simulink subsystem "VehicleElec"  (R2023a)
settings: Solver=VariableStepAuto  StartTime=0.0  StopTime=10.0  RelTol=1e-3
undefined symbols (not defined in the file): battery, cabin_T_init, vehicleThermal
libraries: fl_lib x95, nesl_utility x28, sdl_lib x8, slpidlib x3, simulink x2, EmotorLib x2, BatteryCurrentManagement x1, ee_lib x1
(part 1 of 3)
settings Model: Creator=jjha  LastModifiedBy=jjha
settings OptimizationCC: ReuseModelBlockBuffer=off

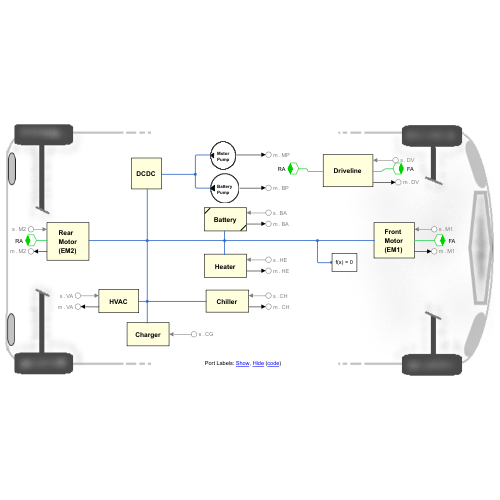
[thumbnail: Simulink's stored preview of the top-level diagram]
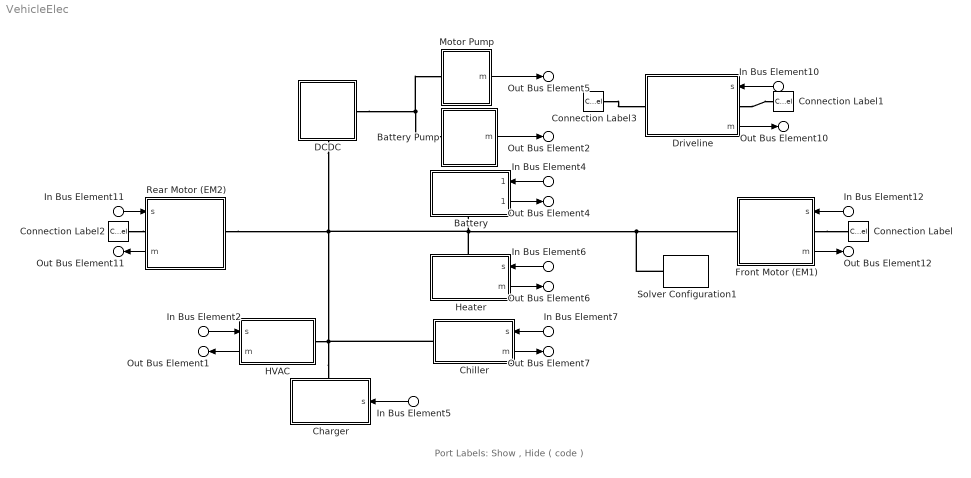
== system VehicleElec ==
  note: Port Labels: Show , Hide ( code )
  In Bus Element2 : Inport  PortName=s  Element=VA
  In Bus Element4 : Inport  PortName=s  Element=BA
  In Bus Element6 : Inport  PortName=s  Element=HE
  In Bus Element7 : Inport  PortName=s  Element=CH
  In Bus Element10 : Inport  PortName=s  Element=DV
  In Bus Element11 : Inport  PortName=s  Element=M2
  In Bus Element12 : Inport  PortName=s  Element=M1
  In Bus Element5 : Inport  PortName=s  Element=CG
  Battery : Subsystem  ReferencedSubsystem=BatteryPlantModelLumped
      settings: PortSchema="{\"entries\":[{\"content\":{\"sides\":[{\"content\":{\"connectorIds\":[\"In1\",\"Out1\"]},\"type\":\"ConnectorPlacement.EquallySpacedRectSide\",\"uuid\":\"8937d0fc-2bf4-4b6f-a857-82b384a76c94\"},{\"content\":{\"side\":\"RIGHT\"},\"type\":\"ConnectorPlacement.EquallySpacedRectSide\",\"uuid\":\"1ccbeec6-a013-4076-9f98-cb308866a19c\"},{\"content\":{\"side\":\"TOP\"},\"type\":\"ConnectorPlacement.EquallySpacedRectSide\",\"uuid\":\"77a454e3-c37c-480e-9dd0-9550186f5eb3\"},{\"content\":{\"connectorIds\":[\"RConn1\"],\"side\":\"BOTTOM\"},\"type\":\"ConnectorPlacement.EquallySpacedRectSide\",\"uuid\":\"f9a87c6a-7374-41c2-a5df-89d60c915a70\"}]},\"type\":\"ConnectorPlacement.EquallySpacedConnector\",\"uuid\":\"fe008494-fd6d-45a8-bf6b-36872afbad95\"}],\"packageUris\":[\"http://schema.mathworks.com/mf0/Connector/R2020b\"],\"version\":\"1.0\"}"
  Battery Pump : Subsystem  Tag=PublishSubsystem
      settings: PortSchema="{\"entries\":[{\"content\":{\"sides\":[{\"content\":{\"connectorIds\":[\"Out1\"]},\"type\":\"ConnectorPlacement.EquallySpacedRectSide\",\"uuid\":\"f321ff85-78a4-45a4-ab97-f20c5abfaf5e\"},{\"content\":{\"connectorIds\":[\"RConn1\"],\"side\":\"RIGHT\"},\"type\":\"ConnectorPlacement.EquallySpacedRectSide\",\"uuid\":\"2baf3540-3ef2-4140-8c68-0a1895e3ee25\"},{\"content\":{\"connectorIds\":[],\"side\":\"TOP\"},\"type\":\"ConnectorPlacement.EquallySpacedRectSide\",\"uuid\":\"1e5b09ba-71c5-41d6-b265-2fb2d783e941\"},{\"content\":{\"connectorIds\":[],\"side\":\"BOTTOM\"},\"type\":\"ConnectorPlacement.EquallySpacedRectSide\",\"uuid\":\"998b9f49-32fc-4a08-8ed4-02bb722e6368\"}]},\"type\":\"ConnectorPlacement.EquallySpacedConnector\",\"uuid\":\"4c01441a-ee4a-4858-900a-4caacc6910c3\"}],\"packageUris\":[\"http://schema.mathworks.com/mf0/Connector/R2020b\"],\"version\":\"1.0\"}"
      mask Display:
      | plot(150*cos(linspace(0, 2*pi, 500)), 150*sin(linspace(0, 2*pi, 500)))
      | patch([-100 -55 -55 -100]-50, [0 24 -24 0], [0 0 0])
      | %disp(get_param(gcb, 'Name'))
      | disp(['{\bf\fontsize{8}' get_param(gcb, 'Name') '}'], 'texmode','on');
  Charger : Subsystem
      settings: PortSchema="{\"entries\":[{\"content\":{\"sides\":[{\"content\":{\"connectorIds\":[\"In1\"]},\"type\":\"ConnectorPlacement.EquallySpacedRectSide\",\"uuid\":\"cb45011f-5d5d-4b7e-92e7-7d115d1e4fd6\"},{\"content\":{\"connectorIds\":[],\"side\":\"RIGHT\"},\"type\":\"ConnectorPlacement.EquallySpacedRectSide\",\"uuid\":\"cd67087d-6bbf-411e-9f50-cc3c1f5fce85\"},{\"content\":{\"connectorIds\":[\"LConn1\"],\"side\":\"TOP\"},\"type\":\"ConnectorPlacement.EquallySpacedRectSide\",\"uuid\":\"32ff64c9-862a-431f-9f24-2baf455cdab5\"}]},\"type\":\"ConnectorPlacement.EquallySpacedConnector\",\"uuid\":\"13ffd7d0-36a1-4766-a9dc-2d010b2a8713\"}],\"packageUris\":[\"http://schema.mathworks.com/mf0/Connector/R2020b\"],\"version\":\"1.0\"}"
      mask Display:
      | %disp(get_param(gcb, 'Name'))
      | disp(['{\bf\fontsize{12}' get_param(gcb, 'Name') '}'], 'texmode','on');
  Chiller : Subsystem
      settings: PortSchema="{\"entries\":[{\"content\":{\"sides\":[{\"content\":{\"connectorIds\":[\"LConn1\"]},\"type\":\"ConnectorPlacement.EquallySpacedRectSide\",\"uuid\":\"5c01cf01-1aa7-4ead-a658-6b31c847d37c\"},{\"content\":{\"connectorIds\":[\"In1\",\"Out1\"],\"side\":\"RIGHT\"},\"type\":\"ConnectorPlacement.EquallySpacedRectSide\",\"uuid\":\"fa598d46-0793-4efa-a9e2-c958f5dfdee6\"},{\"content\":{\"connectorIds\":[],\"side\":\"TOP\"},\"type\":\"ConnectorPlacement.EquallySpacedRectSide\",\"uuid\":\"e82d971a-2580-41ee-87fa-0ab5603b5665\"},{\"content\":{\"connectorIds\":[],\"side\":\"BOTTOM\"},\"type\":\"ConnectorPlacement.EquallySpacedRectSide\",\"uuid\":\"431a910f-738f-40ab-a4d4-f974d0793b92\"}]},\"type\":\"ConnectorPlacement.EquallySpacedConnector\",\"uuid\":\"9f63eeb1-1768-47e0-a5e5-2e43c100d3fd\"}],\"packageUris\":[\"http://schema.mathworks.com/mf0/Connector/R2020b\"],\"version\":\"1.0\"}"
      mask Display:
      | %disp(get_param(gcb, 'Name'))
      | disp(['{\bf\fontsize{12}' get_param(gcb, 'Name') '}'], 'texmode','on');
  Connection Label : ConnectionLabel  Label=FA
  Connection Label1 : ConnectionLabel  Label=FA
  Connection Label2 : ConnectionLabel  Label=RA
  Connection Label3 : ConnectionLabel  Label=RA
  DCDC : Subsystem
      settings: PortSchema="{\"entries\":[{\"content\":{\"sides\":[{\"content\":{\"connectorIds\":[]},\"type\":\"ConnectorPlacement.EquallySpacedRectSide\",\"uuid\":\"88f70306-1074-4a2f-bf6e-5266a6fad5cc\"},{\"content\":{\"connectorIds\":[\"RConn1\"],\"side\":\"RIGHT\"},\"type\":\"ConnectorPlacement.EquallySpacedRectSide\",\"uuid\":\"c9954f31-88d1-45ba-bccc-746174ca97ad\"},{\"content\":{\"connectorIds\":[],\"side\":\"TOP\"},\"type\":\"ConnectorPlacement.EquallySpacedRectSide\",\"uuid\":\"3d242faa-6d27-4f03-9691-d9501eee9202\"},{\"content\":{\"connectorIds\":[\"RConn2\"],\"side\":\"BOTTOM\"},\"type\":\"ConnectorPlacement.EquallySpacedRectSide\",\"uuid\":\"dbc5cd88-c0c4-43cc-b68d-d7b9b93e8ccf\"}]},\"type\":\"ConnectorPlacement.EquallySpacedConnector\",\"uuid\":\"8b73b678-f81c-41f4-a7f6-152147edfd1f\"}],\"packageUris\":[\"http://schema.mathworks.com/mf0/Connector/R2020b\"],\"version\":\"1.0\"}"
      mask Display:
      | %disp(get_param(gcb, 'Name'))
      | disp(['{\bf\fontsize{12}' get_param(gcb, 'Name') '}'], 'texmode','on');
  Driveline : Subsystem
      settings: PortSchema="{\"entries\":[{\"content\":{\"sides\":[{\"content\":{\"connectorIds\":[\"In1\",\"LConn1\",\"Out1\"]},\"type\":\"ConnectorPlacement.EquallySpacedRectSide\",\"uuid\":\"f321ff85-78a4-45a4-ab97-f20c5abfaf5e\"},{\"content\":{\"connectorIds\":[\"RConn1\"],\"side\":\"RIGHT\"},\"type\":\"ConnectorPlacement.EquallySpacedRectSide\",\"uuid\":\"2baf3540-3ef2-4140-8c68-0a1895e3ee25\"},{\"content\":{\"connectorIds\":[],\"side\":\"TOP\"},\"type\":\"ConnectorPlacement.EquallySpacedRectSide\",\"uuid\":\"1e5b09ba-71c5-41d6-b265-2fb2d783e941\"}]},\"type\":\"ConnectorPlacement.EquallySpacedConnector\",\"uuid\":\"4c01441a-ee4a-4858-900a-4caacc6910c3\"}],\"packageUris\":[\"http://schema.mathworks.com/mf0/Connector/R2020b\"],\"version\":\"1.0\"}"
      mask Display:
      | %disp(get_param(gcb, 'Name'))
      | disp(['{\bf\fontsize{12}' get_param(gcb, 'Name') '}'], 'texmode','on');
  Front Motor (EM1) : Subsystem
      settings: PortSchema="{\"entries\":[{\"content\":{\"sides\":[{\"content\":{\"connectorIds\":[\"In1\",\"LConn1\",\"Out1\"]},\"type\":\"ConnectorPlacement.EquallySpacedRectSide\",\"uuid\":\"7243fc6e-711d-4968-986e-a6ac860e50c1\"},{\"content\":{\"connectorIds\":[\"RConn1\"],\"side\":\"RIGHT\"},\"type\":\"ConnectorPlacement.EquallySpacedRectSide\",\"uuid\":\"18479f7a-8f27-458a-ae71-b38762574ae4\"},{\"content\":{\"connectorIds\":[],\"side\":\"TOP\"},\"type\":\"ConnectorPlacement.EquallySpacedRectSide\",\"uuid\":\"aa936f76-6865-41c5-8414-293bd7d656ce\"},{\"content\":{\"connectorIds\":[],\"side\":\"BOTTOM\"},\"type\":\"ConnectorPlacement.EquallySpacedRectSide\",\"uuid\":\"336e35a4-9a9a-4631-a8f5-a4d8b8cf9e70\"}]},\"type\":\"ConnectorPlacement.EquallySpacedConnector\",\"uuid\":\"faab3502-7b69-46ce-a6d2-3155f4c3b486\"}],\"packageUris\":[\"http://schema.mathworks.com/mf0/Connector/R2020b\"],\"version\":\"1.0\"}"
      mask Display:
      | %disp(get_param(gcb, 'Name'))
      | disp(['{\bf\fontsize{12}' get_param(gcb, 'Name') '}'], 'texmode','on');
  HVAC : Subsystem
      settings: PortSchema="{\"entries\":[{\"content\":{\"sides\":[{\"content\":{\"connectorIds\":[\"LConn1\"]},\"type\":\"ConnectorPlacement.EquallySpacedRectSide\",\"uuid\":\"f3199610-b7b9-4772-9d43-f46decbe6ee9\"},{\"content\":{\"connectorIds\":[\"In1\",\"Out1\"],\"side\":\"RIGHT\"},\"type\":\"ConnectorPlacement.EquallySpacedRectSide\",\"uuid\":\"92399d3a-435b-4545-8fb9-2408b0c62154\"},{\"content\":{\"connectorIds\":[],\"side\":\"TOP\"},\"type\":\"ConnectorPlacement.EquallySpacedRectSide\",\"uuid\":\"9d5257be-bcde-46da-a005-cbe35149e50d\"},{\"content\":{\"connectorIds\":[],\"side\":\"BOTTOM\"},\"type\":\"ConnectorPlacement.EquallySpacedRectSide\",\"uuid\":\"da7f19de-1e57-4fc2-b5c3-4c1d680ac086\"}]},\"type\":\"ConnectorPlacement.EquallySpacedConnector\",\"uuid\":\"aa27bbb1-a774-4836-83ea-faf9e12779cd\"}],\"packageUris\":[\"http://schema.mathworks.com/mf0/Connector/R2020b\"],\"version\":\"1.0\"}"
      mask Display:
      | %disp(get_param(gcb, 'Name'))
      | disp(['{\bf\fontsize{12}' get_param(gcb, 'Name') '}'], 'texmode','on');
  Heater : Subsystem
      settings: PortSchema="{\"entries\":[{\"content\":{\"sides\":[{\"content\":{\"connectorIds\":[]},\"type\":\"ConnectorPlacement.EquallySpacedRectSide\",\"uuid\":\"f321ff85-78a4-45a4-ab97-f20c5abfaf5e\"},{\"content\":{\"connectorIds\":[\"RConn1\"],\"side\":\"RIGHT\"},\"type\":\"ConnectorPlacement.EquallySpacedRectSide\",\"uuid\":\"2baf3540-3ef2-4140-8c68-0a1895e3ee25\"},{\"content\":{\"connectorIds\":[\"Out1\",\"In1\"],\"side\":\"TOP\"},\"type\":\"ConnectorPlacement.EquallySpacedRectSide\",\"uuid\":\"1e5b09ba-71c5-41d6-b265-2fb2d783e941\"},{\"content\":{\"connectorIds\":[],\"side\":\"BOTTOM\"},\"type\":\"ConnectorPlacement.EquallySpacedRectSide\",\"uuid\":\"2993c442-350f-4391-ac34-e98798b669d5\"}]},\"type\":\"ConnectorPlacement.EquallySpacedConnector\",\"uuid\":\"4c01441a-ee4a-4858-900a-4caacc6910c3\"}],\"packageUris\":[\"http://schema.mathworks.com/mf0/Connector/R2020b\"],\"version\":\"1.0\"}"
      mask Display:
      | %disp(get_param(gcb, 'Name'))
      | disp(['{\bf\fontsize{12}' get_param(gcb, 'Name') '}'], 'texmode','on');
  Motor Pump : Subsystem  Tag=PublishSubsystem
      settings: PortSchema="{\"entries\":[{\"content\":{\"sides\":[{\"content\":{\"connectorIds\":[\"Out1\"]},\"type\":\"ConnectorPlacement.EquallySpacedRectSide\",\"uuid\":\"dafa5c41-979f-4f2b-beb0-03378b6030c3\"},{\"content\":{\"connectorIds\":[\"RConn1\"],\"side\":\"RIGHT\"},\"type\":\"ConnectorPlacement.EquallySpacedRectSide\",\"uuid\":\"2ea2b4cc-bcb0-4b93-915b-9928efecd2a3\"},{\"content\":{\"connectorIds\":[],\"side\":\"TOP\"},\"type\":\"ConnectorPlacement.EquallySpacedRectSide\",\"uuid\":\"e510a9c0-a763-4750-a71a-9698d7ffd631\"},{\"content\":{\"connectorIds\":[],\"side\":\"BOTTOM\"},\"type\":\"ConnectorPlacement.EquallySpacedRectSide\",\"uuid\":\"6a9cd967-74c4-4a03-9c08-7c7b4b09ecc0\"}]},\"type\":\"ConnectorPlacement.EquallySpacedConnector\",\"uuid\":\"4a878def-b7f5-448f-823c-c871001bb196\"}],\"packageUris\":[\"http://schema.mathworks.com/mf0/Connector/R2020b\"],\"version\":\"1.0\"}"
      mask Display:
      | plot(150*cos(linspace(0, 2*pi, 500)), 150*sin(linspace(0, 2*pi, 500)))
      | patch([-100 -55 -55 -100]-50, [0 24 -24 0], [0 0 0])
      | %disp(get_param(gcb, 'Name'))
      | disp(['{\bf\fontsize{8}' get_param(gcb, 'Name') '}'], 'texmode','on');
  Rear Motor (EM2) : Subsystem
      settings: PortSchema="{\"entries\":[{\"content\":{\"sides\":[{\"content\":{\"connectorIds\":[\"LConn1\"]},\"type\":\"ConnectorPlacement.EquallySpacedRectSide\",\"uuid\":\"50b93907-dab5-4c80-8f3d-b9696f7ba561\"},{\"content\":{\"connectorIds\":[\"In1\",\"RConn1\",\"Out1\"],\"side\":\"RIGHT\"},\"type\":\"ConnectorPlacement.EquallySpacedRectSide\",\"uuid\":\"ca5b0fd2-80b7-4a93-a409-39e052d42ed0\"},{\"content\":{\"connectorIds\":[],\"side\":\"TOP\"},\"type\":\"ConnectorPlacement.EquallySpacedRectSide\",\"uuid\":\"a20c906c-aee3-4b84-9c3f-344dbfe549ed\"},{\"content\":{\"connectorIds\":[],\"side\":\"BOTTOM\"},\"type\":\"ConnectorPlacement.EquallySpacedRectSide\",\"uuid\":\"c8c8c4b4-9dd9-46bd-a7c0-676d6e20cefe\"}]},\"type\":\"ConnectorPlacement.EquallySpacedConnector\",\"uuid\":\"5e07fad4-8c29-4119-b1ea-c96ebc59433e\"}],\"packageUris\":[\"http://schema.mathworks.com/mf0/Connector/R2020b\"],\"version\":\"1.0\"}"
      mask Display:
      | %disp(get_param(gcb, 'Name'))
      | disp(['{\bf\fontsize{12}' get_param(gcb, 'Name') '}'], 'texmode','on');
  Solver Configuration1 : nesl_utility/Solver Configuration  PhysicalDomain=network_engine_domain  SubClassName=solver  LeftPortType=input  RightPortType=generic  Tones=[]  Harmonics=[]  SimulateNoise=off  Profile=off  UseLocalSampling=off  EnableSwitchedLinearOptims=on  FrequencyDomain=off  UseCCode=off  RelTol=0.001  AbsTol=0.001  MinStep=1e-09  ToWorkspace=off  RevertToSquareIcSolve=off  NumHomotopyIterations=100  PhasorMode=off  PhasorModeNumHarmonics=1  ConsistencySolver=NEWTON_XTOL_AFTER_FTOL  IndexReductionMethod=DerivativeReplacement  DoDC=off  ResidualTolerance=1e-09  ConsistencyTolSource=GLOBAL  ConsistencyAbsTol=0.001  ConsistencyRelTol=0.001  ConsistencyTolFactor=0.001  UseLocalSolver=off  LocalSolverChoice=NE_BACKWARD_EULER_ADVANCER  ResolveIndetEquations=on  FunctionEvalNumThread=1  LocalSolverSampleTime=0.001  DoFixedCost=off  MaxNonlinIter=3  MaxModeIter=2  ComputeImpulses=off  ImpulseIterations=2  LinearAlgebra=auto  LinearAlgebraNumThread=0  EquationFormulation=NE_TIME_EF  DelaysMemoryBudget=1024  AutomaticFiltering=on  FilteringTimeConstant=0.001  PartitionStorageMethod=AS_NEEDED  PartitionMemoryBudget=1024  PartitionMethod=ROBUST
  Out Bus Element1 : Outport  PortName=m  Element=VA
  Out Bus Element4 : Outport  PortName=m  Element=BA
  Out Bus Element6 : Outport  PortName=m  Element=HE
  Out Bus Element7 : Outport  PortName=m  Element=CH
  Out Bus Element10 : Outport  PortName=m  Element=DV
  Out Bus Element11 : Outport  PortName=m  Element=M2
  Out Bus Element12 : Outport  PortName=m  Element=M1
  Out Bus Element5 : Outport  PortName=m  Element=MP
  Out Bus Element2 : Outport  PortName=m  Element=BP
  wires:
  In Bus Element2/1 -> HVAC/1(s)
  In Bus Element6/1 -> Heater/1(s)
  In Bus Element4/1 -> Battery/1
  Chiller/1(m) -> Out Bus Element7/1
  In Bus Element7/1 -> Chiller/1(s)
  Battery/1 -> Out Bus Element4/1
  HVAC/1(m) -> Out Bus Element1/1
  Driveline/1(m) -> Out Bus Element10/1
  In Bus Element10/1 -> Driveline/1(s)
  In Bus Element11/1 -> Rear Motor (EM2)/1(s)
  Rear Motor (EM2)/1(m) -> Out Bus Element11/1
  In Bus Element12/1 -> Front Motor (EM1)/1(s)
  Front Motor (EM1)/1(m) -> Out Bus Element12/1
  In Bus Element5/1 -> Charger/1(s)
  Heater/1(m) -> Out Bus Element6/1
  Motor Pump/1("  m ") -> Out Bus Element5/1
  Battery Pump/1("  m ") -> Out Bus Element2/1
  connections:
  Charger/LConn1 -- Solver Configuration1/RConn1 -- Front Motor (EM1)/RConn1 -- Heater/RConn1 -- Battery/RConn1 -- DCDC/RConn2 -- Rear Motor (EM2)/LConn1 -- HVAC/LConn1 -- Chiller/LConn1
  Battery Pump/RConn1 -- DCDC/RConn1 -- Motor Pump/RConn1
  Connection Label2/LConn1 -- Rear Motor (EM2)/RConn1
  Front Motor (EM1)/LConn1 -- Connection Label/LConn1
  Driveline/LConn1 -- Connection Label1/LConn1
  Connection Label3/LConn1 -- Driveline/RConn1

== system VehicleElec/Battery Pump ==
  Controlled Current Source : fl_lib/Electrical/Electrical Sources/Controlled Current Source
  Electrical Reference : fl_lib/Electrical/Electrical Elements/Electrical Reference
  PS Constant : fl_lib/Physical Signals/Sources/PS Constant  constant=0 A
  current sensing1 : Subsystem
      settings: PortSchema="{\"entries\":[{\"content\":{\"sides\":[{\"content\":{\"connectorIds\":[\"LConn1\"]},\"type\":\"ConnectorPlacement.EquallySpacedRectSide\",\"uuid\":\"be2815b5-7c4b-4452-9f46-9765620d338b\"},{\"content\":{\"connectorIds\":[\"RConn1\"],\"side\":\"RIGHT\"},\"type\":\"ConnectorPlacement.EquallySpacedRectSide\",\"uuid\":\"398ebab2-f4fa-4d00-bf6e-74bf1f6972c5\"},{\"content\":{\"connectorIds\":[\"Out1\"],\"side\":\"TOP\"},\"type\":\"ConnectorPlacement.EquallySpacedRectSide\",\"uuid\":\"f18d5713-17ec-4be9-9072-3e03c5a4f599\"}]},\"type\":\"ConnectorPlacement.EquallySpacedConnector\",\"uuid\":\"966ec05e-6316-4039-8e26-1d6b096cf423\"}],\"packageUris\":[\"http://schema.mathworks.com/mf0/Connector/R2020b\"],\"version\":\"1.0\"}"
  LV : PMIOPort  Side=Right
  Bus Element Out : Outport  PortName=m  Element=BattPumpCurr
  wires:
  current sensing1/1("   ") -> Bus Element Out/1  "BattPumpCurr"
  connections:
  Controlled Current Source/LConn1 -- Electrical Reference/LConn1
  PS Constant/RConn1 -- Controlled Current Source/RConn1
  current sensing1/RConn1 -- Controlled Current Source/RConn2
  current sensing1/LConn1 -- LV/RConn1

== system VehicleElec/Charger ==
  s : Inport
  Battery CC-CV : BatteryCurrentManagement/Battery CC-CV  MaxCellVoltage=battery.ChargeMaxVolt  Kp=battery.ChargeKp  Ki=battery.ChargerKi  Kaw=battery.ChargerKaw  Kt=1  Ts=-1
      settings: LibrarySourceBlock=batt_sl_lib/Current Management/Battery CC-CV
  Bus Selector4 : BusSelector  OutputSignals=Batt.Relay.RelayChg,Batt.BattSensor.CellVoltMax
  Constant Chg Current : Constant  Value=battery.ChargerCC_A
  Controlled Current Source : fl_lib/Electrical/Electrical Sources/Controlled Current Source
  Electrical Reference : fl_lib/Electrical/Electrical Elements/Electrical Reference
  Ground : Ground
  Simulink-PS Converter1 : nesl_utility/Simulink-PS Converter  PhysicalDomain=network_engine_domain  SubClassName=ps_input  LeftPortType=input  RightPortType=output  PseudoPeriodic=off  Frequencies=[]  NoiseDistribution=none  NoiseParameters=[]  Unit=A  AffineConversion=off  FilteringAndDerivatives=filter  SimscapeFilterOrder=2  InputFilterTimeConstant=0.01  UdotUserProvided=0
  Transfer Fcn : TransferFcn  Denominator=[1 1]
  HV : PMIOPort  Side=Left
  wires:
  Transfer Fcn/1 -> Simulink-PS Converter1/1
  Constant Chg Current/1 -> Battery CC-CV/3
  Bus Selector4/2 -> Battery CC-CV/2  "<CellVoltMax>"
  Bus Selector4/1 -> Battery CC-CV/1  "<RelayChg>"
  Battery CC-CV/1 -> Transfer Fcn/1
  Ground/1 -> Battery CC-CV/4
  s/1 -> Bus Selector4/1
  connections:
  Electrical Reference/LConn1 -- Controlled Current Source/RConn2
  HV/RConn1 -- Controlled Current Source/LConn1
  Controlled Current Source/RConn1 -- Simulink-PS Converter1/RConn1

== system VehicleElec/Chiller ==
  s : Inport
  Bus Selector : BusSelector  OutputSignals=Batt.BatSt,cmdChillerByp
  Chiller Subsystem : Subsystem
      settings: PortSchema="{\"entries\":[{\"content\":{\"sides\":[{\"content\":{\"connectorIds\":[\"LConn1\",\"In1\",\"In2\"]},\"type\":\"ConnectorPlacement.EquallySpacedRectSide\",\"uuid\":\"d995acd0-973b-4873-b050-eaa71c2c53f5\"},{\"content\":{\"connectorIds\":[\"RConn1\",\"RConn2\"],\"side\":\"RIGHT\"},\"type\":\"ConnectorPlacement.EquallySpacedRectSide\",\"uuid\":\"f40dc2d9-a9a2-427c-8e3f-65ba63c73559\"},{\"content\":{\"connectorIds\":[],\"side\":\"TOP\"},\"type\":\"ConnectorPlacement.EquallySpacedRectSide\",\"uuid\":\"1868aaf5-b9f5-4fdb-94e9-4b9189d403a5\"}]},\"type\":\"ConnectorPlacement.EquallySpacedConnector\",\"uuid\":\"c13a0ccf-549d-47cf-8e66-a96ce55255c8\"}],\"packageUris\":[\"http://schema.mathworks.com/mf0/Connector/R2020b\"],\"version\":\"1.0\"}"
  Controlled Current Source : fl_lib/Electrical/Electrical Sources/Controlled Current Source
  Electrical Reference : fl_lib/Electrical/Electrical Elements/Electrical Reference
  Electrical Reference1 : fl_lib/Electrical/Electrical Elements/Electrical Reference
  PS Terminator : fl_lib/Physical Signals/Sinks/PS Terminator
  Voltage Sensor : fl_lib/Electrical/Electrical Sensors/Voltage Sensor
  current sensing1 : Subsystem
      settings: PortSchema="{\"entries\":[{\"content\":{\"sides\":[{\"content\":{\"connectorIds\":[\"LConn1\"]},\"type\":\"ConnectorPlacement.EquallySpacedRectSide\",\"uuid\":\"be2815b5-7c4b-4452-9f46-9765620d338b\"},{\"content\":{\"connectorIds\":[\"RConn1\"],\"side\":\"RIGHT\"},\"type\":\"ConnectorPlacement.EquallySpacedRectSide\",\"uuid\":\"398ebab2-f4fa-4d00-bf6e-74bf1f6972c5\"},{\"content\":{\"connectorIds\":[\"Out1\"],\"side\":\"TOP\"},\"type\":\"ConnectorPlacement.EquallySpacedRectSide\",\"uuid\":\"f18d5713-17ec-4be9-9072-3e03c5a4f599\"}]},\"type\":\"ConnectorPlacement.EquallySpacedConnector\",\"uuid\":\"966ec05e-6316-4039-8e26-1d6b096cf423\"}],\"packageUris\":[\"http://schema.mathworks.com/mf0/Connector/R2020b\"],\"version\":\"1.0\"}"
  HV : PMIOPort  Side=Left
  Bus Element Out : Outport  PortName=m  Element=ChillerCurrent
  wires:
  s/1 -> Bus Selector/1
  current sensing1/1("   ") -> Bus Element Out/1  "AuxHiCurrentC"
  Bus Selector/2 -> Chiller Subsystem/2(ThCtrl)  "<cmdChillerByp>"
  Bus Selector/1 -> Chiller Subsystem/1(BattSt)  "<BatSt>"
  connections:
  Voltage Sensor/RConn1 -- Chiller Subsystem/LConn1
  Electrical Reference1/LConn1 -- Voltage Sensor/RConn2
  Controlled Current Source/RConn1 -- Chiller Subsystem/RConn1
  Controlled Current Source/LConn1 -- Electrical Reference/LConn1
  HV/RConn1 -- Voltage Sensor/LConn1 -- current sensing1/LConn1
  Controlled Current Source/RConn2 -- current sensing1/RConn1
  PS Terminator/LConn1 -- Chiller Subsystem/RConn2

== system VehicleElec/DCDC ==
  DC-DC Converter : ee_lib/Semiconductors & Converters/Converters/DC-DC Converter  Vref_option=ee.enum.converters.voltageref.internal  v_ref=100 V  P_rated=10000 W  droop_enabled=false  droop_param=ee.enum.converters.droop.value  droop=0.1 V/A  droop_percent=2  Vref_droop=10 V  reversible=ee.enum.converters.directionality.unidirectional  G_diode=1e-8 1/Ohm  P_fixed=1 W  losses_option=ee.enum.converters.lossesOption.proportionalToSquaredCurrent  eff_rated=80  tableOption=ee.enum.converters.lossTableOptionThermal.currentTemp  i_eff_vec=[-2, -1, 1, 2] A  v_eff_vec=[15, 30, 45] V  eff_vec=[66, 76, 80, 74]  eff_2D_table=[66, 66, 66; 76, 76, 76; 80, 80, 80; 74, 74, 74]  model_dynamics=ee.enum.converters.dynamics.yes  tau=0.02 s  v_ini=10 V  v1_min=1 V  R1=1000 Ohm  R2=1000 Ohm  enable_fault=simscape.enum.onoff.off  fault_condition=ee.enum.faults.faultInputCondition.greaterThan  fault_threshold=0.5  T_eff_vec=[280, 300, 320] K  eff_3D_table=repmat([66; 76; 80; 74], 1, 3, 3)  thermal_mass=100 J/K  initial_temperature=298.15 K
      settings: InternalSimscapePortConfiguration="{\"Bottom\":[],\"Left\":[{\"id\":\"p1\",\"label\":\"1+\",\"type\":\"foundation.electrical.electrical\"},{\"id\":\"n1\",\"label\":\"1-\",\"type\":\"foundation.electrical.electrical\"}],\"Right\":[{\"id\":\"p2\",\"label\":\"2+\",\"type\":\"foundation.electrical.electrical\"},{\"id\":\"n2\",\"label\":\"2-\",\"type\":\"foundation.electrical.electrical\"}],\"Top\":[]}"
  Electrical Reference : fl_lib/Electrical/Electrical Elements/Electrical Reference
  Electrical Reference1 : fl_lib/Electrical/Electrical Elements/Electrical Reference
  LV : PMIOPort  Side=Right
  HV : PMIOPort  Port=2  Side=Right
  connections:
  LV/RConn1 -- DC-DC Converter/RConn1
  Electrical Reference/LConn1 -- DC-DC Converter/RConn2
  HV/RConn1 -- DC-DC Converter/LConn1
  DC-DC Converter/LConn2 -- Electrical Reference1/LConn1

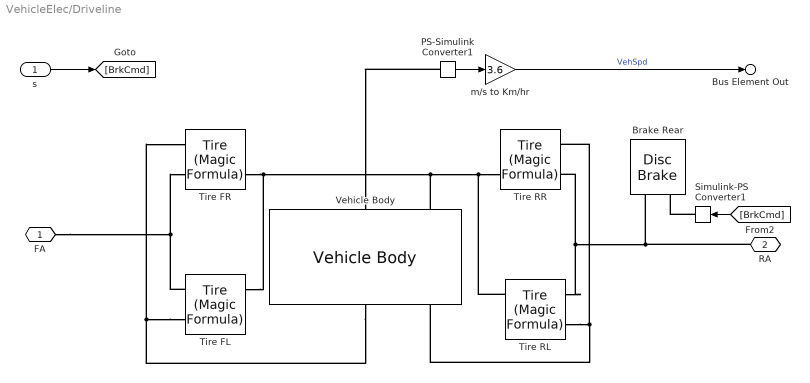
== system VehicleElec/Driveline ==
  s : Inport
  Brake Rear : sdl_lib/Brakes & Detents/Rotational/Disc Brake  r_mean=150 mm  bore=10 mm  n_pads=2  thermal_port=simscape.enum.thermaleffects.omit  mu_static=0.9  mu_coulomb=0.7  temperature_TLU=[280, 300, 320] K  mu_static_TLU=[.9, .8, .7]  mu_coulomb_TLU=[.8, .7, .6]  brkwy_vel=0.1 rad/s  visc_coef=0 N*m*s/rad  enable_faults=simscape.enum.onoff.off  faulted_pressure=0 bar  external_fault=simscape.enum.onoff.off  temporal_fault=simscape.enum.onoff.off  fault_time=5 s  report_fault=simscape.enum.assert.action.none  thermal_mass=50 kJ/K  temperature_specify=off  temperature_priority=High  temperature=300 K  temperature_nominal_specify=off  temperature_nominal_unit=K  temperature_nominal_value=1
  PS-Simulink Converter1 : nesl_utility/PS-Simulink Converter  PhysicalDomain=network_engine_domain  SubClassName=ps_output  LeftPortType=input  RightPortType=output  PseudoPeriodic=off  Frequencies=[]  VectorFormat=inherit  Unit=inherit  AffineConversion=off
  Simulink-PS Converter1 : nesl_utility/Simulink-PS Converter  PhysicalDomain=network_engine_domain  SubClassName=ps_input  LeftPortType=input  RightPortType=output  PseudoPeriodic=off  Frequencies=[]  NoiseDistribution=none  NoiseParameters=[]  Unit=1  AffineConversion=off  FilteringAndDerivatives=provide  SimscapeFilterOrder=1  InputFilterTimeConstant=0.001  UdotUserProvided=0
  Tire FL : sdl_lib/Tires & Vehicles/Tire (Magic Formula)  parameterization=sdl.enum.magic_tire_model.peak  F_z1=3000 N  F_x1=3500 N  kappa1=10  B_m=10  C_m=1.9  D_m=1  E_m=0.97  fz0=4000 N  p_Cx=1.685  p_Dx=[1.21, -.037]  p_Ex=[.344, .095, -.02, 0]  p_Kx=[21.51, -.163, .245]  p_Hx=[-.002, .002]  p_Vx=[0, 0]  rolling_radius_model=sdl.enum.RollingRadiusParameterization.Constant  r_e="vehicle.tireRollingRadius_cm  cm"  r_0=0.3 m  breff=8.39  dreff=0.26  freff=0.074  q_re0=0.99  q_v1=0.008  longvl=17 m/s  cz=5e5 N/m  model_resistance=simscape.enum.onoff.off  resistance_model=sdl.enum.rollingResistanceParameterization.constant  coeff=0.015  p_tire=250e3 Pa  alpha=-0.003  beta=0.97  coeff_a=84e-4  coeff_b=6.2e-4 s/m  coeff_c=1.6e-4 s^2/m^2  p_tire0=240e3 Pa  fz0_resistance=4000 N  vH0=16 m/s  q_Sy=[.0082, 0, .0014, .001, 0, 0, 1.08, -.5]  v_thr=0.001 m/s  enable_scaling_coefficients=false  lfzO=1  lcx=1  lmux=1  lex=1  lkx=1  lhx=1  lvx=1  lmy=1  model_compliance=sdl.enum.compliance.off  stiffness=1e6 N/m  damping=1000 N*s/m  model_inertia=sdl.enum.model_inertia.off  inertia=1 kg*m^2  initial_velocity=0 rad/s  vxlow=0.1 m/s  v_tr_thr=0.1*(0.1) m/s  kpumin=-1e5  kpumax=1e5
  Tire FR : sdl_lib/Tires & Vehicles/Tire (Magic Formula)  parameterization=sdl.enum.magic_tire_model.peak  F_z1=3000 N  F_x1=3500 N  kappa1=10  B_m=10  C_m=1.9  D_m=1  E_m=0.97  fz0=4000 N  p_Cx=1.685  p_Dx=[1.21, -.037]  p_Ex=[.344, .095, -.02, 0]  p_Kx=[21.51, -.163, .245]  p_Hx=[-.002, .002]  p_Vx=[0, 0]  rolling_radius_model=sdl.enum.RollingRadiusParameterization.Constant  r_e="vehicle.tireRollingRadius_cm  cm"  r_0=0.3 m  breff=8.39  dreff=0.26  freff=0.074  q_re0=0.99  q_v1=0.008  longvl=17 m/s  cz=5e5 N/m  model_resistance=simscape.enum.onoff.off  resistance_model=sdl.enum.rollingResistanceParameterization.constant  coeff=0.015  p_tire=250e3 Pa  alpha=-0.003  beta=0.97  coeff_a=84e-4  coeff_b=6.2e-4 s/m  coeff_c=1.6e-4 s^2/m^2  p_tire0=240e3 Pa  fz0_resistance=4000 N  vH0=16 m/s  q_Sy=[.0082, 0, .0014, .001, 0, 0, 1.08, -.5]  v_thr=0.001 m/s  enable_scaling_coefficients=false  lfzO=1  lcx=1  lmux=1  lex=1  lkx=1  lhx=1  lvx=1  lmy=1  model_compliance=sdl.enum.compliance.off  stiffness=1e6 N/m  damping=1000 N*s/m  model_inertia=sdl.enum.model_inertia.off  inertia=1 kg*m^2  initial_velocity=0 rad/s  vxlow=0.1 m/s  v_tr_thr=0.1*(0.1) m/s  kpumin=-1e5  kpumax=1e5
  Tire RL : sdl_lib/Tires & Vehicles/Tire (Magic Formula)  parameterization=sdl.enum.magic_tire_model.peak  F_z1=3000 N  F_x1=3500 N  kappa1=10  B_m=10  C_m=1.9  D_m=1  E_m=0.97  fz0=4000 N  p_Cx=1.685  p_Dx=[1.21, -.037]  p_Ex=[.344, .095, -.02, 0]  p_Kx=[21.51, -.163, .245]  p_Hx=[-.002, .002]  p_Vx=[0, 0]  rolling_radius_model=sdl.enum.RollingRadiusParameterization.Constant  r_e="vehicle.tireRollingRadius_cm  cm"  r_0=0.3 m  breff=8.39  dreff=0.26  freff=0.074  q_re0=0.99  q_v1=0.008  longvl=17 m/s  cz=5e5 N/m  model_resistance=simscape.enum.onoff.off  resistance_model=sdl.enum.rollingResistanceParameterization.constant  coeff=0.015  p_tire=250e3 Pa  alpha=-0.003  beta=0.97  coeff_a=84e-4  coeff_b=6.2e-4 s/m  coeff_c=1.6e-4 s^2/m^2  p_tire0=240e3 Pa  fz0_resistance=4000 N  vH0=16 m/s  q_Sy=[.0082, 0, .0014, .001, 0, 0, 1.08, -.5]  v_thr=0.001 m/s  enable_scaling_coefficients=false  lfzO=1  lcx=1  lmux=1  lex=1  lkx=1  lhx=1  lvx=1  lmy=1  model_compliance=sdl.enum.compliance.off  stiffness=1e6 N/m  damping=1000 N*s/m  model_inertia=sdl.enum.model_inertia.off  inertia=1 kg*m^2  initial_velocity=0 rad/s  vxlow=0.1 m/s  v_tr_thr=0.1*(0.1) m/s  kpumin=-1e5  kpumax=1e5
  Tire RR : sdl_lib/Tires & Vehicles/Tire (Magic Formula)  parameterization=sdl.enum.magic_tire_model.peak  F_z1=3000 N  F_x1=3500 N  kappa1=10  B_m=10  C_m=1.9  D_m=1  E_m=0.97  fz0=4000 N  p_Cx=1.685  p_Dx=[1.21, -.037]  p_Ex=[.344, .095, -.02, 0]  p_Kx=[21.51, -.163, .245]  p_Hx=[-.002, .002]  p_Vx=[0, 0]  rolling_radius_model=sdl.enum.RollingRadiusParameterization.Constant  r_e="vehicle.tireRollingRadius_cm  cm"  r_0=0.3 m  breff=8.39  dreff=0.26  freff=0.074  q_re0=0.99  q_v1=0.008  longvl=17 m/s  cz=5e5 N/m  model_resistance=simscape.enum.onoff.off  resistance_model=sdl.enum.rollingResistanceParameterization.constant  coeff=0.015  p_tire=250e3 Pa  alpha=-0.003  beta=0.97  coeff_a=84e-4  coeff_b=6.2e-4 s/m  coeff_c=1.6e-4 s^2/m^2  p_tire0=240e3 Pa  fz0_resistance=4000 N  vH0=16 m/s  q_Sy=[.0082, 0, .0014, .001, 0, 0, 1.08, -.5]  v_thr=0.001 m/s  enable_scaling_coefficients=false  lfzO=1  lcx=1  lmux=1  lex=1  lkx=1  lhx=1  lvx=1  lmy=1  model_compliance=sdl.enum.compliance.off  stiffness=1e6 N/m  damping=1000 N*s/m  model_inertia=sdl.enum.model_inertia.off  inertia=1 kg*m^2  initial_velocity=0 rad/s  vxlow=0.1 m/s  v_tr_thr=0.1*(0.1) m/s  kpumin=-1e5  kpumax=1e5
  Vehicle Body : sdl_lib/Tires & Vehicles/Vehicle Body  mass=vehicle.vehMass_kg kg  n_w=2  x_f=1.4 m  x_r=1.6 m  y_c=0.5 m  mass_var=simscape.enum.onoff.off  g=9.81 m/s^2  liftoff_warning=simscape.enum.onoff.off  area=3 m^2  Cd=0.4  rho=1.18 kg/m^3  model_pitch=simscape.enum.onoff.off  inertia=4000 kg*m^2  suspension_model=sdl.enum.linearTLU.linear  k_f=1e4 N/m  b_f=1e4 N*s/m  k_r=1e4 N/m  b_r=1e4 N*s/m  k_f_TLU=[-2000, -1000, 0, 1000, 2000] N  x_f_TLU=[-.4, -.2, 0, .2, .4] m  b_f_TLU=[-200, -100, 0, 100, 200] N  v_f_TLU=[-4, -2, 0, 2, 4] m/s  k_r_TLU=[-2000, -1000, 0, 1000, 2000] N  x_r_TLU=[-.4, -.2, 0, .2, .4] m  b_r_TLU=[-200, -100, 0, 100, 200] N  v_r_TLU=[-4, -2, 0, 2, 4] m/s  interp_method=simscape.enum.interpolation.linear  extrap_method=simscape.enum.extrapolation.linear  model_hardstop=simscape.enum.onoff.off  upper_bound_f=.25 m  lower_bound_f=-.25 m  stop_k_f=1e6 N/m  stop_b_f=150 N*s/m  upper_bound_r=.25 m  lower_bound_r=-.25 m  stop_k_r=1e6 N/m  stop_b_r=150 N*s/m  initial_pitch=0 rad  initial_pitch_rate=0 rad/s  v_specify=on  v_priority=High  v=0 kph  v_nominal_specify=on  v_nominal_unit=m/s  v_nominal_value=1
  m/s to Km/hr : Gain  Gain=3.6
  FA : PMIOPort  Side=Left
  RA : PMIOPort  Port=2  Side=Right
  Bus Element Out : Outport  PortName=m  Element=VehSpd
  wires:
  s/1 -> [BrkCmd]
  PS-Simulink Converter1/1 -> m/s to Km/hr/1
  m/s to Km/hr/1 -> Bus Element Out/1  "VehSpd"
  [BrkCmd] -> Simulink-PS Converter1/1
  connections:
  Tire FL/LConn1 -- Tire FR/LConn1 -- Vehicle Body/RConn2
  Tire RR/LConn1 -- Vehicle Body/RConn1 -- Tire RL/LConn1
  PS-Simulink Converter1/LConn1 -- Vehicle Body/LConn2
  Tire FR/LConn2 -- FA/RConn1 -- Tire FL/LConn2
  Brake Rear/LConn2 -- RA/RConn1 -- Tire RR/LConn2 -- Tire RL/LConn2
  Tire FL/RConn2 -- Vehicle Body/LConn1 -- Tire RR/RConn2 -- Tire RL/RConn2 -- Tire FR/RConn2
  Simulink-PS Converter1/RConn1 -- Brake Rear/LConn1

== system VehicleElec/Front Motor (EM1) ==
  s : Inport
  Bus Creator : BusCreator  Inputs=3
  Bus Selector : BusSelector  OutputSignals=EM1Trq,Batt
  Constant : Constant  Value=293
  Emotor : EmotorLib/Emotor  max_torque=electricDrive.max_torque  max_power=electricDrive.max_power  Tctc=electricDrive.Tctc  spMat=electricDrive.motor_loss_map.spMat  tqMat=electricDrive.motor_loss_map.tqMat  lossMat=electricDrive.motor_loss_map.lossMat
  Emotor Input : Subsystem
  Emotor Output : Subsystem
  Gear : sdl_lib/Gears/Simple Gear  ratio=10/3  rotation_direction=sdl.enum.shaftOutputDirection.same  friction_model=sdl.enum.gear_efficiencies_load.off  T_noload=0.1 N*m  T_nom=5 N*m  efficiency_nom=0.8  efficiency=0.8  temperature_TLU=[280, 300, 320] K  load_TLU=[1, 5, 10] N*m  efficiency_TLU=[.95, .9, .85]  efficiency_TLU2=[.85, .8, .75; .95, .9, .85; .85, .8, .7]  w_thr=0.01 rad/s  pwr_thr=0.001 W  enable_backlash=false  hardstop_model=simscape.enum.hardstop.smooth  backlash_distance=1e-3 mm  r_base=0.1 m  transition=1e-4 mm  backlash_stiffness=1e7 N/m  backlash_damping=1e6 N*s/m  coeff_rest=0  v_tol=0.001 m/s  f_tol=0 N  mu_visc=[0, 0] N*m*s/rad  enable_faults=simscape.enum.onoff.off  efficiency_fault=0.05  external_fault=simscape.enum.onoff.off  temporal_fault=simscape.enum.onoff.off  fault_time=5 s  fault_angles=pi / 12 rad  report_fault=simscape.enum.assert.action.none  thermal_mass=50 J/K  temperature_specify=off  temperature_priority=High  temperature=300 K  temperature_nominal_specify=off  temperature_nominal_unit=K  temperature_nominal_value=1  x_backlash_specify=off  x_backlash_priority=None  x_backlash=0 mm  x_backlash_nominal_specify=off  x_backlash_nominal_unit=mm  x_backlash_nominal_value=1  f_hardstop_specify=off  f_hardstop_priority=None  f_hardstop=0 N  f_hardstop_nominal_specify=off  f_hardstop_nominal_unit=N  f_hardstop_nominal_value=1  v_backlash_specify=off  v_backlash_priority=None  v_backlash=0 m/s  v_backlash_nominal_specify=off  v_backlash_nominal_unit=m/s  v_backlash_nominal_value=1
  Ax : PMIOPort  Side=Left
  HV : PMIOPort  Port=2  Side=Right
  m : Outport
  wires:
  s/1 -> Bus Selector/1
  Bus Creator/1 -> m/1
  Constant/1 -> Bus Creator/3  "CoolTp"
  Emotor Output/2(E) -> Bus Creator/2  "EMenergy"
  Emotor Output/1(EM) -> Bus Creator/1  "EM"
  Emotor/1 -> Emotor Output/1(S)
  Emotor Input/1(EMctl) -> Emotor/1
  Bus Selector/2 -> Emotor Input/2("Batt ")  "<Batt>"
  Bus Selector/1 -> Emotor Input/1("Tq  ")  "<EM1Trq>"
  connections:
  Emotor/LConn1 -- HV/RConn1
  Emotor/RConn1 -- Gear/LConn1
  Gear/RConn1 -- Ax/RConn1

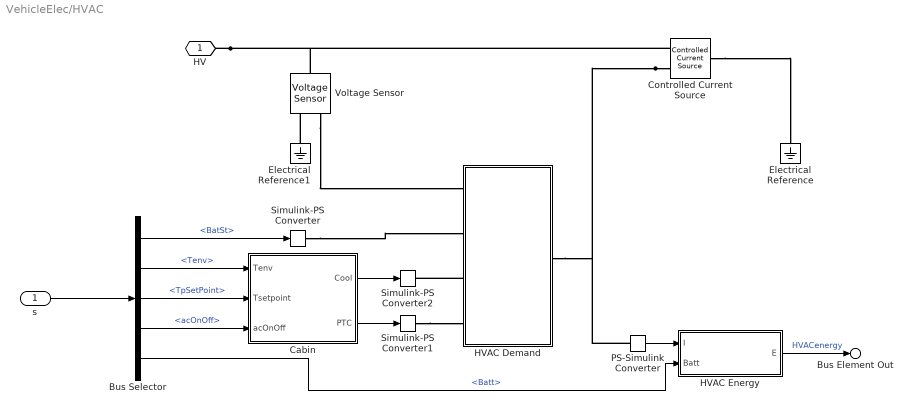
== system VehicleElec/HVAC ==
  s : Inport
  Bus Selector : BusSelector  OutputSignals=Batt.BatSt,Tenv,TpSetPoint,acOnOff,Batt
  Cabin : Subsystem
  Controlled Current Source : fl_lib/Electrical/Electrical Sources/Controlled Current Source
  Electrical Reference : fl_lib/Electrical/Electrical Elements/Electrical Reference
  Electrical Reference1 : fl_lib/Electrical/Electrical Elements/Electrical Reference
  HVAC Demand : Subsystem
  HVAC Energy : Subsystem
  PS-Simulink Converter : nesl_utility/PS-Simulink Converter  PhysicalDomain=network_engine_domain  SubClassName=ps_output  LeftPortType=input  RightPortType=output  PseudoPeriodic=off  Frequencies=[]  VectorFormat=inherit  Unit=inherit  AffineConversion=off
  Simulink-PS Converter : nesl_utility/Simulink-PS Converter  PhysicalDomain=network_engine_domain  SubClassName=ps_input  LeftPortType=input  RightPortType=output  PseudoPeriodic=off  Frequencies=[]  NoiseDistribution=none  NoiseParameters=[]  Unit=1  AffineConversion=off  FilteringAndDerivatives=provide  SimscapeFilterOrder=1  InputFilterTimeConstant=0.001  UdotUserProvided=0
  Simulink-PS Converter1 : nesl_utility/Simulink-PS Converter  PhysicalDomain=network_engine_domain  SubClassName=ps_input  LeftPortType=input  RightPortType=output  PseudoPeriodic=off  Frequencies=[]  NoiseDistribution=none  NoiseParameters=[]  Unit=W  AffineConversion=off  FilteringAndDerivatives=provide  SimscapeFilterOrder=1  InputFilterTimeConstant=0.001  UdotUserProvided=0
  Simulink-PS Converter2 : nesl_utility/Simulink-PS Converter  PhysicalDomain=network_engine_domain  SubClassName=ps_input  LeftPortType=input  RightPortType=output  PseudoPeriodic=off  Frequencies=[]  NoiseDistribution=none  NoiseParameters=[]  Unit=W  AffineConversion=off  FilteringAndDerivatives=provide  SimscapeFilterOrder=1  InputFilterTimeConstant=0.001  UdotUserProvided=0
  Voltage Sensor : fl_lib/Electrical/Electrical Sensors/Voltage Sensor
  HV : PMIOPort  Side=Left
  Bus Element Out : Outport  PortName=m  Element=HVACenergy
  wires:
  Bus Selector/1 -> Simulink-PS Converter/1  "<BatSt>"
  Cabin/2(PTC) -> Simulink-PS Converter1/1
  Cabin/1(Cool) -> Simulink-PS Converter2/1
  Bus Selector/5 -> HVAC Energy/2(Batt)  "<Batt>"
  PS-Simulink Converter/1 -> HVAC Energy/1(I)
  Bus Selector/4 -> Cabin/3(acOnOff)  "<acOnOff>"
  Bus Selector/3 -> Cabin/2(Tsetpoint)  "<TpSetPoint>"
  Bus Selector/2 -> Cabin/1(Tenv)  "<Tenv>"
  s/1 -> Bus Selector/1
  HVAC Energy/1(E) -> Bus Element Out/1  "HVACenergy"
  connections:
  Controlled Current Source/RConn1 -- PS-Simulink Converter/LConn1 -- HVAC Demand/RConn1
  Simulink-PS Converter1/RConn1 -- HVAC Demand/LConn4
  HVAC Demand/LConn3 -- Simulink-PS Converter2/RConn1
  Simulink-PS Converter/RConn1 -- HVAC Demand/LConn2
  Voltage Sensor/RConn1 -- HVAC Demand/LConn1
  Electrical Reference1/LConn1 -- Voltage Sensor/RConn2
  HV/RConn1 -- Voltage Sensor/LConn1 -- Controlled Current Source/RConn2
  Controlled Current Source/LConn1 -- Electrical Reference/LConn1

== system VehicleElec/Heater ==
  s : Inport
  Bus Selector : BusSelector  OutputSignals=BatSt,cmdHeater
  Controlled Current Source : fl_lib/Electrical/Electrical Sources/Controlled Current Source
  Electrical Reference : fl_lib/Electrical/Electrical Elements/Electrical Reference
  Electrical Reference1 : fl_lib/Electrical/Electrical Elements/Electrical Reference
  Heater Subsystem : Subsystem
      settings: PortSchema="{\"entries\":[{\"content\":{\"sides\":[{\"content\":{\"connectorIds\":[\"LConn1\",\"In1\",\"In2\"]},\"type\":\"ConnectorPlacement.EquallySpacedRectSide\",\"uuid\":\"d995acd0-973b-4873-b050-eaa71c2c53f5\"},{\"content\":{\"connectorIds\":[\"RConn1\",\"RConn2\"],\"side\":\"RIGHT\"},\"type\":\"ConnectorPlacement.EquallySpacedRectSide\",\"uuid\":\"f40dc2d9-a9a2-427c-8e3f-65ba63c73559\"},{\"content\":{\"connectorIds\":[],\"side\":\"TOP\"},\"type\":\"ConnectorPlacement.EquallySpacedRectSide\",\"uuid\":\"1868aaf5-b9f5-4fdb-94e9-4b9189d403a5\"}]},\"type\":\"ConnectorPlacement.EquallySpacedConnector\",\"uuid\":\"c13a0ccf-549d-47cf-8e66-a96ce55255c8\"}],\"packageUris\":[\"http://schema.mathworks.com/mf0/Connector/R2020b\"],\"version\":\"1.0\"}"
  PS Terminator : fl_lib/Physical Signals/Sinks/PS Terminator
  Voltage Sensor : fl_lib/Electrical/Electrical Sensors/Voltage Sensor
  current sensing1 : Subsystem
      settings: PortSchema="{\"entries\":[{\"content\":{\"sides\":[{\"content\":{\"connectorIds\":[\"LConn1\"]},\"type\":\"ConnectorPlacement.EquallySpacedRectSide\",\"uuid\":\"be2815b5-7c4b-4452-9f46-9765620d338b\"},{\"content\":{\"connectorIds\":[\"RConn1\"],\"side\":\"RIGHT\"},\"type\":\"ConnectorPlacement.EquallySpacedRectSide\",\"uuid\":\"398ebab2-f4fa-4d00-bf6e-74bf1f6972c5\"},{\"content\":{\"connectorIds\":[\"Out1\"],\"side\":\"TOP\"},\"type\":\"ConnectorPlacement.EquallySpacedRectSide\",\"uuid\":\"f18d5713-17ec-4be9-9072-3e03c5a4f599\"}]},\"type\":\"ConnectorPlacement.EquallySpacedConnector\",\"uuid\":\"966ec05e-6316-4039-8e26-1d6b096cf423\"}],\"packageUris\":[\"http://schema.mathworks.com/mf0/Connector/R2020b\"],\"version\":\"1.0\"}"
  HV : PMIOPort  Side=Right
  Bus Element Out : Outport  PortName=m  Element=HeaterCurrent
  wires:
  s/1 -> Bus Selector/1
  Bus Selector/2 -> Heater Subsystem/2(ThCtrl)  "<cmdHeater>"
  Bus Selector/1 -> Heater Subsystem/1(Batt)  "<BatSt>"
  current sensing1/1("   ") -> Bus Element Out/1  "AuxHiCurrentH"
  connections:
  Voltage Sensor/RConn1 -- Heater Subsystem/LConn1
  Electrical Reference1/LConn1 -- Voltage Sensor/RConn2
  Controlled Current Source/RConn1 -- Heater Subsystem/RConn1
  Controlled Current Source/LConn1 -- Electrical Reference/LConn1
  HV/RConn1 -- Voltage Sensor/LConn1 -- current sensing1/LConn1
  Controlled Current Source/RConn2 -- current sensing1/RConn1
  PS Terminator/LConn1 -- Heater Subsystem/RConn2

== system VehicleElec/Motor Pump ==
  Controlled Current Source : fl_lib/Electrical/Electrical Sources/Controlled Current Source
  Electrical Reference : fl_lib/Electrical/Electrical Elements/Electrical Reference
  Electrical Reference1 : fl_lib/Electrical/Electrical Elements/Electrical Reference
  PS Constant : fl_lib/Physical Signals/Sources/PS Constant  constant=0 A
  PS-Simulink Converter2 : nesl_utility/PS-Simulink Converter  PhysicalDomain=network_engine_domain  SubClassName=ps_output  LeftPortType=input  RightPortType=output  PseudoPeriodic=off  Frequencies=[]  VectorFormat=inherit  Unit=inherit  AffineConversion=off
  Voltage Sensor : fl_lib/Electrical/Electrical Sensors/Voltage Sensor
  current sensing : Subsystem
      settings: PortSchema="{\"entries\":[{\"content\":{\"sides\":[{\"content\":{\"connectorIds\":[\"LConn1\"]},\"type\":\"ConnectorPlacement.EquallySpacedRectSide\",\"uuid\":\"be2815b5-7c4b-4452-9f46-9765620d338b\"},{\"content\":{\"connectorIds\":[\"RConn1\"],\"side\":\"RIGHT\"},\"type\":\"ConnectorPlacement.EquallySpacedRectSide\",\"uuid\":\"398ebab2-f4fa-4d00-bf6e-74bf1f6972c5\"},{\"content\":{\"connectorIds\":[\"Out1\"],\"side\":\"TOP\"},\"type\":\"ConnectorPlacement.EquallySpacedRectSide\",\"uuid\":\"f18d5713-17ec-4be9-9072-3e03c5a4f599\"}]},\"type\":\"ConnectorPlacement.EquallySpacedConnector\",\"uuid\":\"966ec05e-6316-4039-8e26-1d6b096cf423\"}],\"packageUris\":[\"http://schema.mathworks.com/mf0/Connector/R2020b\"],\"version\":\"1.0\"}"
  LV : PMIOPort  Side=Right
  Bus Element Out : Outport  PortName=m  Element=MotorPumpCurr
  Bus Element Out1 : Outport  PortName=m  Element=LowVolt
  wires:
  current sensing/1("   ") -> Bus Element Out/1  "MotorPumpCurr"
  PS-Simulink Converter2/1 -> Bus Element Out1/1
  connections:
  PS Constant/RConn1 -- Controlled Current Source/RConn1
  Electrical Reference1/LConn1 -- Voltage Sensor/RConn2
  Voltage Sensor/RConn1 -- PS-Simulink Converter2/LConn1
  Controlled Current Source/LConn1 -- Electrical Reference/LConn1
  Controlled Current Source/RConn2 -- current sensing/RConn1
  LV/RConn1 -- current sensing/LConn1 -- Voltage Sensor/LConn1

== system VehicleElec/Rear Motor (EM2) ==
  s : Inport
  Bus Creator : BusCreator  Inputs=3
  Bus Selector : BusSelector  OutputSignals=EM2Trq,Batt
  Constant : Constant  Value=293
  Emotor : EmotorLib/Emotor  max_torque=electricDrive.max_torque  max_power=electricDrive.max_power  Tctc=electricDrive.Tctc  spMat=electricDrive.motor_loss_map.spMat  tqMat=electricDrive.motor_loss_map.tqMat  lossMat=electricDrive.motor_loss_map.lossMat
  Emotor Input : Subsystem
  Emotor Output : Subsystem
  Gear : sdl_lib/Gears/Simple Gear  ratio=10/3  rotation_direction=sdl.enum.shaftOutputDirection.same  friction_model=sdl.enum.gear_efficiencies_load.off  T_noload=0.1 N*m  T_nom=5 N*m  efficiency_nom=0.8  efficiency=0.8  temperature_TLU=[280, 300, 320] K  load_TLU=[1, 5, 10] N*m  efficiency_TLU=[.95, .9, .85]  efficiency_TLU2=[.85, .8, .75; .95, .9, .85; .85, .8, .7]  w_thr=0.01 rad/s  pwr_thr=0.001 W  enable_backlash=false  hardstop_model=simscape.enum.hardstop.smooth  backlash_distance=1e-3 mm  r_base=0.1 m  transition=1e-4 mm  backlash_stiffness=1e7 N/m  backlash_damping=1e6 N*s/m  coeff_rest=0  v_tol=0.001 m/s  f_tol=0 N  mu_visc=[0, 0] N*m*s/rad  enable_faults=simscape.enum.onoff.off  efficiency_fault=0.05  external_fault=simscape.enum.onoff.off  temporal_fault=simscape.enum.onoff.off  fault_time=5 s  fault_angles=pi / 12 rad  report_fault=simscape.enum.assert.action.none  thermal_mass=50 J/K  temperature_specify=off  temperature_priority=High  temperature=300 K  temperature_nominal_specify=off  temperature_nominal_unit=K  temperature_nominal_value=1  x_backlash_specify=off  x_backlash_priority=None  x_backlash=0 mm  x_backlash_nominal_specify=off  x_backlash_nominal_unit=mm  x_backlash_nominal_value=1  f_hardstop_specify=off  f_hardstop_priority=None  f_hardstop=0 N  f_hardstop_nominal_specify=off  f_hardstop_nominal_unit=N  f_hardstop_nominal_value=1  v_backlash_specify=off  v_backlash_priority=None  v_backlash=0 m/s  v_backlash_nominal_specify=off  v_backlash_nominal_unit=m/s  v_backlash_nominal_value=1
  HV : PMIOPort  Side=Left
  Ax : PMIOPort  Port=2  Side=Right
  m : Outport
  wires:
  Constant/1 -> Bus Creator/3  "CoolTp"
  s/1 -> Bus Selector/1
  Emotor Output/2(E) -> Bus Creator/2  "EMenergy"
  Emotor Output/1(EM2) -> Bus Creator/1  "EM"
  Bus Creator/1 -> m/1
  Emotor Input/1(EMctl) -> Emotor/1
  Emotor/1 -> Emotor Output/1(S)
  Bus Selector/2 -> Emotor Input/2(" Batt")  "<Batt>"
  Bus Selector/1 -> Emotor Input/1(TrqCmd)  "<EM2Trq>"
  connections:
  HV/RConn1 -- Emotor/LConn1
  Ax/RConn1 -- Gear/RConn1
  Gear/LConn1 -- Emotor/RConn1

== system VehicleElec/Battery Pump/current sensing1 ==
  Current Sensor : fl_lib/Electrical/Electrical Sensors/Current Sensor
  PS-Simulink Converter : nesl_utility/PS-Simulink Converter  PhysicalDomain=network_engine_domain  SubClassName=ps_output  LeftPortType=input  RightPortType=output  PseudoPeriodic=off  Frequencies=[]  VectorFormat=inherit  Unit=inherit  AffineConversion=off
  "  " : PMIOPort  Side=Left
  " " : PMIOPort  Port=2  Side=Right
  "   " : Outport
  wires:
  PS-Simulink Converter/1 -> "   "/1
  connections:
  Current Sensor/RConn2 -- " "/RConn1
  Current Sensor/LConn1 -- "  "/RConn1
  PS-Simulink Converter/LConn1 -- Current Sensor/RConn1

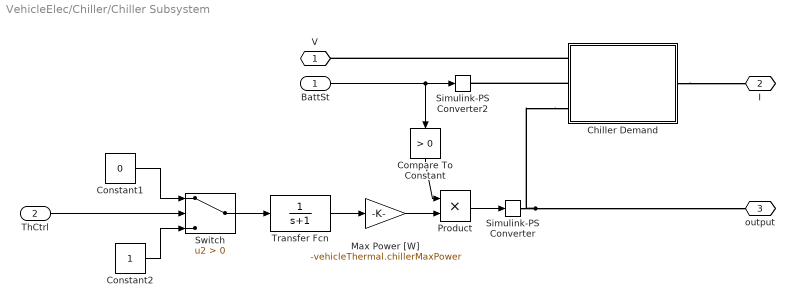
== system VehicleElec/Chiller/Chiller Subsystem ==
  BattSt : Inport
  ThCtrl : Inport  Port=2
  Chiller Demand : Subsystem
  Compare To Constant : simulink/Logic and Bit Operations/Compare To Constant  relop=>  const=0  OutDataTypeStr=boolean
  Constant1 : Constant  Value=0
  Constant2 : Constant
  Max Power [W] : Gain  Gain=-vehicleThermal.chillerMaxPower
  Product : Product
  Simulink-PS Converter : nesl_utility/Simulink-PS Converter  PhysicalDomain=network_engine_domain  SubClassName=ps_input  LeftPortType=input  RightPortType=output  PseudoPeriodic=off  Frequencies=[]  NoiseDistribution=none  NoiseParameters=[]  Unit=W  AffineConversion=off  FilteringAndDerivatives=provide  SimscapeFilterOrder=1  InputFilterTimeConstant=0.001  UdotUserProvided=0
  Simulink-PS Converter2 : nesl_utility/Simulink-PS Converter  PhysicalDomain=network_engine_domain  SubClassName=ps_input  LeftPortType=input  RightPortType=output  PseudoPeriodic=off  Frequencies=[]  NoiseDistribution=none  NoiseParameters=[]  Unit=1  AffineConversion=off  FilteringAndDerivatives=provide  SimscapeFilterOrder=1  InputFilterTimeConstant=0.001  UdotUserProvided=0
  Switch : Switch  Criteria=u2 > Threshold  SaturateOnIntegerOverflow=off  InputSameDT=off
  Transfer Fcn : TransferFcn  Denominator=[1 1]
  V : PMIOPort  Side=Left
  I : PMIOPort  Port=2  Side=Right
  output : PMIOPort  Port=3  Side=Right
  wires:
  Constant1/1 -> Switch/1
  Constant2/1 -> Switch/3
  Compare To Constant/1 -> Product/1
  Product/1 -> Simulink-PS Converter/1
  BattSt/1 -> Simulink-PS Converter2/1, Compare To Constant/1
  Transfer Fcn/1 -> Max Power [W]/1
  ThCtrl/1 -> Switch/2
  Switch/1 -> Transfer Fcn/1
  Max Power [W]/1 -> Product/2
  connections:
  Chiller Demand/RConn1 -- I/RConn1
  Chiller Demand/LConn2 -- Simulink-PS Converter2/RConn1
  Chiller Demand/LConn1 -- V/RConn1
  Chiller Demand/LConn3 -- output/RConn1 -- Simulink-PS Converter/RConn1

== system VehicleElec/Chiller/current sensing1 ==
  Current Sensor : fl_lib/Electrical/Electrical Sensors/Current Sensor
  PS-Simulink Converter : nesl_utility/PS-Simulink Converter  PhysicalDomain=network_engine_domain  SubClassName=ps_output  LeftPortType=input  RightPortType=output  PseudoPeriodic=off  Frequencies=[]  VectorFormat=inherit  Unit=inherit  AffineConversion=off
  "  " : PMIOPort  Side=Left
  " " : PMIOPort  Port=2  Side=Right
  "   " : Outport
  wires:
  PS-Simulink Converter/1 -> "   "/1
  connections:
  Current Sensor/RConn2 -- " "/RConn1
  Current Sensor/LConn1 -- "  "/RConn1
  PS-Simulink Converter/LConn1 -- Current Sensor/RConn1

== system VehicleElec/Front Motor (EM1)/Emotor Input ==
  "Tq  " : Inport
  "Batt " : Inport  Port=2
  Bus Creator : BusCreator  Inputs=3
  Bus Selector3 : BusSelector  OutputSignals=Relay.RelayDchg,BattSensor.BatVolt
  Constant : Constant
  Constant1 : Constant  Value=0
  Gain : Gain
  Switch : Switch  Criteria=u2 > Threshold  SaturateOnIntegerOverflow=off  InputSameDT=off
  EMctl : Outport
  wires:
  Gain/1 -> Bus Creator/3  "BatVolt"
  Bus Selector3/2 -> Gain/1  "<BatVolt>"
  Bus Creator/1 -> EMctl/1
  "Batt "/1 -> Bus Selector3/1
  Bus Selector3/1 -> Switch/2  "<RelayDchg>"
  Constant/1 -> Switch/3
  Constant1/1 -> Switch/1
  Switch/1 -> Bus Creator/2  "fault"
  "Tq  "/1 -> Bus Creator/1  "EMtrq"

== system VehicleElec/Front Motor (EM1)/Emotor Output ==
  S : Inport
  Bus Selector1 : BusSelector  OutputSignals=Current,Volt
  Constant : Constant  Value=3600
  Divide : Product  Inputs=*/
  Integrator : Integrator
  Product : Product
  EM : Outport
  E : Outport  Port=2
  wires:
  Bus Selector1/1 -> Product/1  "<Current>"
  Bus Selector1/2 -> Product/2  "<Volt>"
  S/1 -> Bus Selector1/1, EM/1  "EMsensor"
  Product/1 -> Integrator/1
  Integrator/1 -> Divide/1
  Constant/1 -> Divide/2
  Divide/1 -> E/1  "EMenergy"

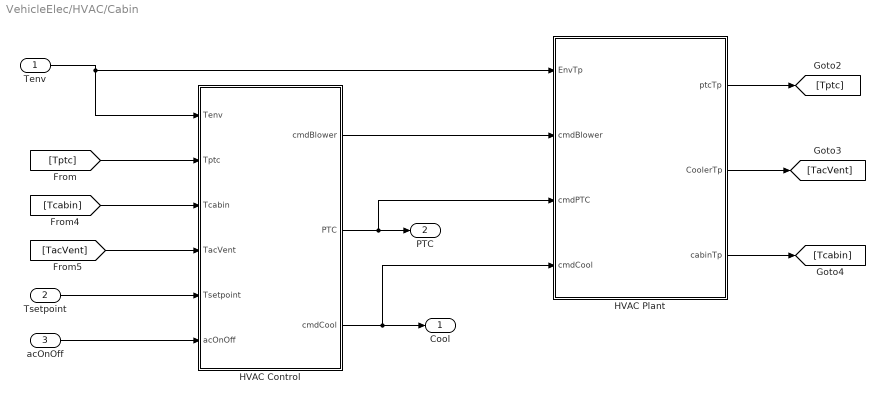
== system VehicleElec/HVAC/Cabin ==
  Tenv : Inport
  Tsetpoint : Inport  Port=2
  acOnOff : Inport  Port=3
  HVAC Control : Subsystem
  HVAC Plant : Subsystem
  Cool : Outport
  PTC : Outport  Port=2
  wires:
  acOnOff/1 -> HVAC Control/6(acOnOff)
  Tenv/1 -> HVAC Plant/1(EnvTp), HVAC Control/1(Tenv)
  Tsetpoint/1 -> HVAC Control/5(Tsetpoint)
  [Tcabin] -> HVAC Control/3(Tcabin)
  [TacVent] -> HVAC Control/4(TacVent)
  HVAC Control/3(cmdCool) -> Cool/1, HVAC Plant/4(cmdCool)
  [Tptc] -> HVAC Control/2(Tptc)
  HVAC Plant/3(cabinTp) -> [Tcabin]
  HVAC Plant/2(CoolerTp) -> [TacVent]
  HVAC Control/1(cmdBlower) -> HVAC Plant/2(cmdBlower)
  HVAC Control/2(PTC) -> HVAC Plant/3(cmdPTC), PTC/1
  HVAC Plant/1(ptcTp) -> [Tptc]
